simulink model "Short_Period_Longitudinal_Motion6"  (R2018b)
settings: Solver=ode4  StartTime=0.0  StopTime=30  FixedStep=0.001  RelTol=1e-3
libraries: simulink x4
settings Model: Creator=aiham  LastModifiedBy=PC 650

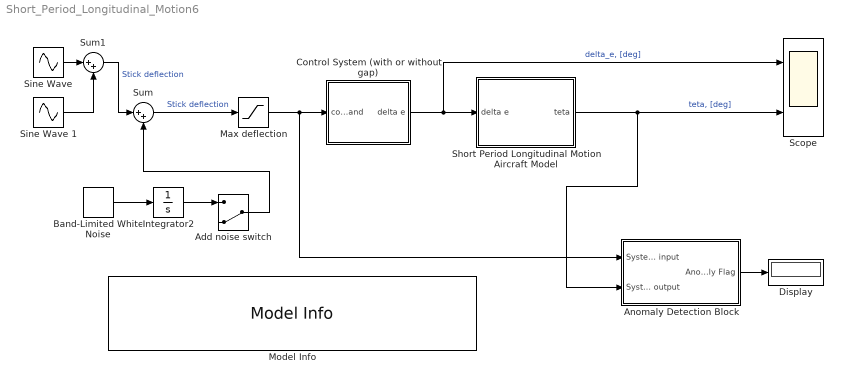
== system Short_Period_Longitudinal_Motion6 ==
  Add noise switch : ManualSwitch  CurrentSetting=0
  Anomaly Detection Block : Subsystem
  "Band-Limited White Noise " : simulink/Sources/Band-Limited White Noise  Cov=[0.01]  Ts=0.1  seed=[23341]
  Control System (with or without gap) : Subsystem
  Display : Display
  Integrator2 : Integrator
  Max deflection : Saturate  UpperLimit=25 / 57.3  LowerLimit=-25 / 57.3
  Model Info : simulink/Model-Wide Utilities/Model Info  Frame=on  DisplayStringWithTags=|  HorizontalTextAlignment=Center  LeftAlignmentValue=0.5
      | Anomaly Detection in Control System
      | using simple Short Period Longitidunal Motion Model 
      | Input: Pilot Stick Deflection, [deg]
      | Output:  Aircraft Pitch Angle, [deg]
      | Anomaly type: Mechanical Gap (Dead Zone) in the longitudinal control system)
  Scope : Scope  NumInputPorts=2
  Short Period Longitudinal Motion Aircraft Model : Subsystem
  "Sine Wave " : Sin  Amplitude="12  / 57.3"  Frequency=pi  Phase=3.1415/4  SampleTime=0
  Sine Wave 1 : Sin  Amplitude=13 / 57.3  Frequency=pi/2  Phase=3*3.1415/2  SampleTime=0
  Sum : Sum  Inputs=|++
  Sum1 : Sum  Inputs=|++
  wires:
  Short Period Longitudinal Motion Aircraft Model/1(teta) -> Scope/2, Anomaly Detection Block/2(System output)  "teta, [deg]"
  Control System (with or without gap)/1(delta e) -> Scope/1, Short Period Longitudinal Motion Aircraft Model/1(delta e)  "delta_e, [deg]"
  "Band-Limited White Noise "/1 -> Integrator2/1
  Integrator2/1 -> Add noise switch/1
  Add noise switch/1 -> Sum/2
  Sum/1 -> Max deflection/1  "Stick deflection"
  Anomaly Detection Block/1(Anomaly Flag) -> Display/1
  Max deflection/1 -> Anomaly Detection Block/1(System input), Control System (with or without gap)/1(command)
  "Sine Wave "/1 -> Sum1/1
  Sum1/1 -> Sum/1  "Stick deflection"
  Sine Wave 1/1 -> Sum1/2

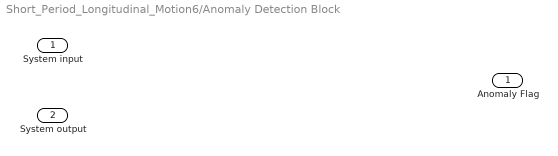
== system Short_Period_Longitudinal_Motion6/Anomaly Detection Block ==
  System input : Inport
  System output : Inport  Port=2
  Anomaly Flag : Outport

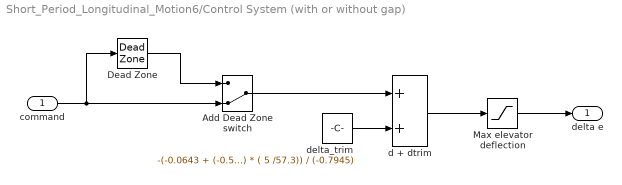
== system Short_Period_Longitudinal_Motion6/Control System (with or without gap) ==
  command : Inport
  Add Dead Zone switch : ManualSwitch  CurrentSetting=0
  "Dead Zone " : DeadZone  LowerValue=-0.02  UpperValue=0.02  SaturateOnIntegerOverflow=on
  Max elevator deflection : Saturate  UpperLimit=25 / 57.3  LowerLimit=-25 / 57.3
  d + dtrim : Sum
  delta_trim : Constant  Value=-(-0.0643 + (-0.5235) * ( 5 /57.3)) / (-0.7945)
  delta e : Outport
  wires:
  delta_trim/1 -> d + dtrim/2
  Add Dead Zone switch/1 -> d + dtrim/1
  d + dtrim/1 -> Max elevator deflection/1
  "Dead Zone "/1 -> Add Dead Zone switch/1
  command/1 -> "Dead Zone "/1, Add Dead Zone switch/2
  Max elevator deflection/1 -> delta e/1

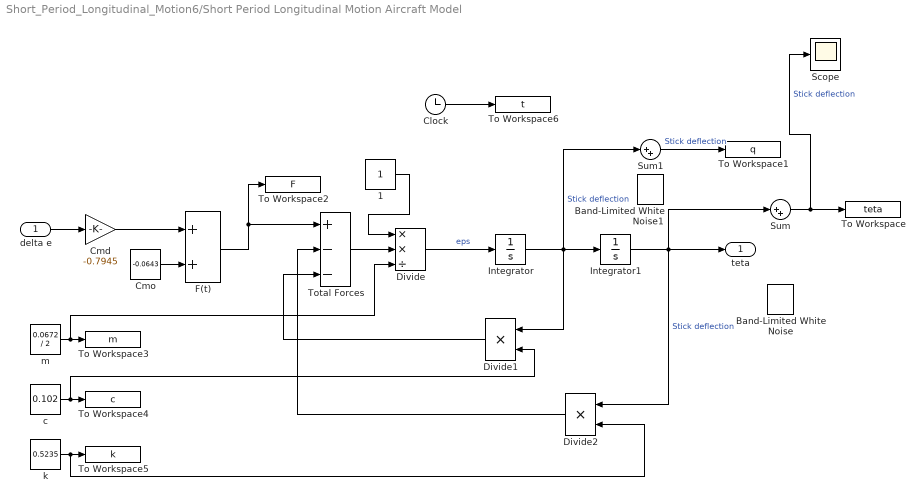
== system Short_Period_Longitudinal_Motion6/Short Period Longitudinal Motion Aircraft Model ==
  delta e : Inport
  1 : Constant
  Band-Limited White Noise : simulink/Sources/Band-Limited White Noise  Cov=[0.001]  Ts=0.1  seed=[23341]
  Band-Limited White Noise1 : simulink/Sources/Band-Limited White Noise  Cov=[0.001]  Ts=0.1  seed=[23341]
  Clock : Clock
  Cmd : Gain  Gain=-0.7945
  Cmo : Constant  Value=-0.0643
  Divide : Product  Inputs=**/
  Divide1 : Product  Inputs=**
  Divide2 : Product  Inputs=**
  F(t) : Sum
  Integrator : Integrator
  Integrator1 : Integrator  InitialCondition=5 / 57.3
  Scope : Scope
  Sum : Sum  Inputs=|++
  Sum1 : Sum  Inputs=|++
  To Workspace : ToWorkspace  VariableName=teta  SampleTime=0.05
  To Workspace1 : ToWorkspace  VariableName=q  SampleTime=0.05
  To Workspace2 : ToWorkspace  VariableName=F  SampleTime=0.05
  To Workspace3 : ToWorkspace  VariableName=m  SampleTime=0.05
      settings: MaxDataPoints=1
  To Workspace4 : ToWorkspace  VariableName=c  SampleTime=0.05
      settings: MaxDataPoints=1
  To Workspace5 : ToWorkspace  VariableName=k  SampleTime=0.05
      settings: MaxDataPoints=1
  To Workspace6 : ToWorkspace  VariableName=t  SampleTime=0.05
  Total Forces : Sum  Inputs=+--
  c : Constant  Value=0.102
  k : Constant  Value=0.5235
  m : Constant  Value=0.0672 / 2
  teta : Outport
  wires:
  Divide1/1 -> Total Forces/3
  Cmo/1 -> F(t)/2
  F(t)/1 -> To Workspace2/1, Total Forces/1
  Divide2/1 -> Total Forces/2
  delta e/1 -> Cmd/1
  Cmd/1 -> F(t)/1
  Total Forces/1 -> Divide/2
  Divide/1 -> Integrator/1  "eps"
  c/1 -> Divide1/2, To Workspace4/1
  k/1 -> Divide2/2, To Workspace5/1
  m/1 -> Divide/3, To Workspace3/1
  1/1 -> Divide/1
  Clock/1 -> To Workspace6/1
  Integrator1/1 -> Sum/1, teta/1, Divide2/1  "Stick deflection"
  Integrator/1 -> Sum1/1, Divide1/1, Integrator1/1  "Stick deflection"
  Sum/1 -> Scope/1, To Workspace/1  "Stick deflection"
  Sum1/1 -> To Workspace1/1  "Stick deflection"
